simulink model "ODE_neurospora_model_leloup"  (R2015a)
settings: Solver=ode4  StartTime=0.0  StopTime=72  FixedStep=0.01  RelTol=1e-3
values from neighbouring files (symbols this model uses):
  daynight_on = 0    [ALL_neurospora_init.m]    (also in ALL_neurospora_sim_run.m; FUZZY_deg_neurospora_init.m; FUZZY_deg_neurospora_sim_run.m; FUZZY_tsc_neurospora_init.m)
  k_1 = 0.5    [ALL_neurospora_init.m]    (also in FUZZY_deg_neurospora_init.m; FUZZY_tsc_neurospora_init.m; FUZZY_tsc_tsl_neurospora_init.m; FUZZY_tsl_neurospora_init.m)
  k_2 = 0.6    [ALL_neurospora_init.m]    (also in FUZZY_deg_neurospora_init.m; FUZZY_tsc_neurospora_init.m; FUZZY_tsc_tsl_neurospora_init.m; FUZZY_tsl_neurospora_init.m)
  K_d = 0.13    [ALL_neurospora_init.m]    (also in FUZZY_deg_neurospora_init.m; FUZZY_tsc_neurospora_init.m; FUZZY_tsc_tsl_neurospora_init.m; FUZZY_tsl_neurospora_init.m)
  K_I = 1    [ALL_neurospora_init.m]    (also in FUZZY_deg_neurospora_init.m; FUZZY_tsc_neurospora_init.m; FUZZY_tsc_tsl_neurospora_init.m; FUZZY_tsl_neurospora_init.m)
  K_m = 0.5    [ALL_neurospora_init.m]    (also in FUZZY_deg_neurospora_init.m; FUZZY_tsc_neurospora_init.m; FUZZY_tsc_tsl_neurospora_init.m; FUZZY_tsl_neurospora_init.m)
  k_s = 0.5    [ALL_neurospora_init.m]    (also in FUZZY_deg_neurospora_init.m; FUZZY_tsc_neurospora_init.m; FUZZY_tsc_tsl_neurospora_init.m; FUZZY_tsl_neurospora_init.m)
  n = 4    [ALL_neurospora_init.m]    (also in FUZZY_deg_neurospora_init.m; FUZZY_tsc_neurospora_init.m; FUZZY_tsc_tsl_neurospora_init.m; FUZZY_tsl_neurospora_init.m)
  v_d = 1.4    [ALL_neurospora_init.m]    (also in FUZZY_deg_neurospora_init.m; FUZZY_tsc_neurospora_init.m; FUZZY_tsc_tsl_neurospora_init.m; FUZZY_tsl_neurospora_init.m)
  v_m = 0.505    [ALL_neurospora_init.m]    (also in FUZZY_deg_neurospora_init.m; FUZZY_tsc_neurospora_init.m; FUZZY_tsc_tsl_neurospora_init.m; FUZZY_tsl_neurospora_init.m)
settings Model: Creator=jureb  LastModifiedBy=jureb

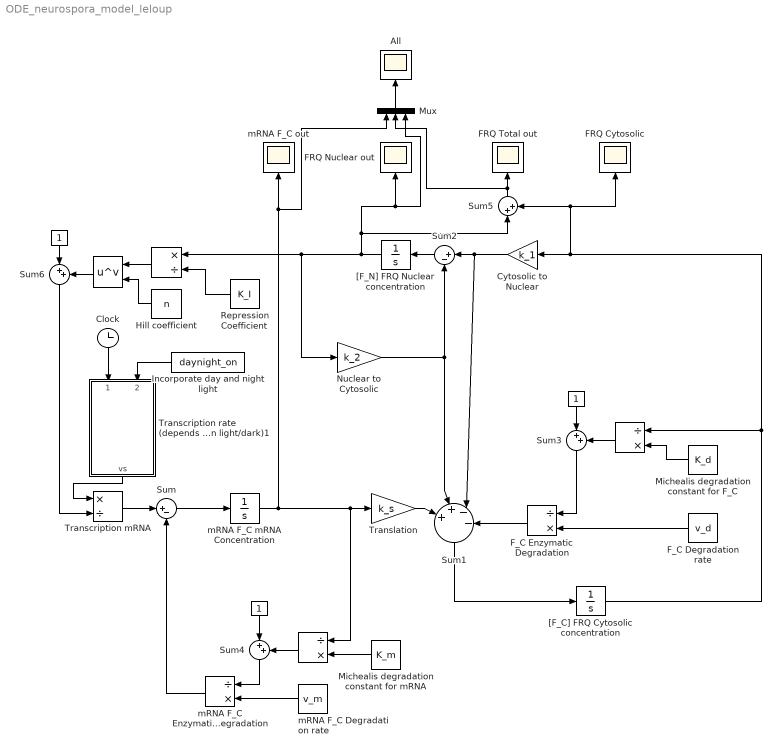
== system ODE_neurospora_model_leloup ==
  " " : Math  Operator=pow  SaturateOnIntegerOverflow=on
  " " : Product  Inputs=/*
  " " : Product  Inputs=*/
  "          " : Constant
  " " : Constant
  " " : Constant
  " " : Product  Inputs=/*
  All : Scope
      settings: TimeRange=71.999776  YMin=0  YMax=9  SaveName=All
  Clock : Clock
  Cytosolic to Nuclear : Gain  Gain=k_1
  FRQ Cytosolic : Scope
      settings: TimeRange=71.999776  YMin=0.5  YMax=10  SaveName=FC_ODE
  FRQ Nuclear out : Scope
      settings: TimeRange=71.999776  YMin=0  YMax=4.5  SaveName=F_N
  FRQ Total out : Scope
      settings: TimeRange=71.999776  YMin=0.5  YMax=10  SaveName=F_ODE
  F_C Degradation rate : Constant  Value=v_d
  F_C Enzymatic Degradation : Product  Inputs=/*
  Hill coefficient : Constant  Value=n
  Incorporate day and night light : Constant  Value=daynight_on
  Michealis degradation constant for F_C : Constant  Value=K_d
  Michealis degradation constant for mRNA : Constant  Value=K_m
  Mux : Mux  Inputs=3
  Nuclear to Cytosolic : Gain  Gain=k_2
  Repression Coefficient : Constant  Value=K_I
  Sum : Sum  Inputs=|+-
  Sum1 : Sum  Inputs=|+|+|-|-
  Sum2 : Sum  Inputs=|+-
  Sum{3..6} (4 alike) : Sum  Inputs=|++
  Transcription mRNA : Product  Inputs=*/
  Transcription rate (depends on light/dark)1 : MATLAB Function  TreatAsAtomicUnit=on
  Translation : Gain  Gain=k_s
  "[F_C] FRQ Cytosolic concentration " : Integrator  InitialCondition=1
  "[F_N] FRQ Nuclear concentration" : Integrator  InitialCondition=1
  mRNA F_C Degradation rate : Constant  Value=v_m
  mRNA F_C Enzymatic Degradation : Product  Inputs=/*
  mRNA F_C mRNA Concentration : Integrator  InitialCondition=1
  mRNA F_C out : Scope
      settings: TimeRange=71.999776  YMin=0  YMax=6  SaveName=mRNA
  wires:
  Sum6/1 -> Transcription mRNA/2
  "          "/1 -> Sum6/1
  " "/1 -> Sum6/2
  Hill coefficient/1 -> " "/2
  Sum/1 -> mRNA F_C mRNA Concentration/1
  " "/1 -> " "/1
  mRNA F_C mRNA Concentration/1 -> Mux/1, mRNA F_C out/1, " "/1, Translation/1
  mRNA F_C Enzymatic Degradation/1 -> Sum/2
  "[F_N] FRQ Nuclear concentration"/1 -> " "/1, Nuclear to Cytosolic/1, Mux/3, FRQ Nuclear out/1, Sum5/1
  Repression Coefficient/1 -> " "/2
  Sum1/1 -> "[F_C] FRQ Cytosolic concentration "/1
  Cytosolic to Nuclear/1 -> Sum1/3, Sum2/1
  Sum2/1 -> "[F_N] FRQ Nuclear concentration"/1
  Nuclear to Cytosolic/1 -> Sum1/2, Sum2/2
  mRNA F_C Degradation rate/1 -> mRNA F_C Enzymatic Degradation/2
  " "/1 -> Sum4/1
  " "/1 -> Sum4/2
  Michealis degradation constant for mRNA/1 -> " "/2
  Sum4/1 -> mRNA F_C Enzymatic Degradation/1
  "[F_C] FRQ Cytosolic concentration "/1 -> FRQ Cytosolic/1, Sum5/2, Cytosolic to Nuclear/1, " "/1
  F_C Enzymatic Degradation/1 -> Sum1/4
  F_C Degradation rate/1 -> F_C Enzymatic Degradation/2
  " "/1 -> Sum3/1
  " "/1 -> Sum3/2
  Michealis degradation constant for F_C/1 -> " "/2
  Sum3/1 -> F_C Enzymatic Degradation/1
  Translation/1 -> Sum1/1
  Mux/1 -> All/1
  Clock/1 -> Transcription rate (depends on light/dark)1/1(sim_time)
  Transcription rate (depends on light/dark)1/1(vs) -> Transcription mRNA/1
  Incorporate day and night light/1 -> Transcription rate (depends on light/dark)1/2(daynight_on)
  Sum5/1 -> Mux/2, FRQ Total out/1
  Transcription mRNA/1 -> Sum/1

== matlab function ODE_neurospora_model_leloup/Transcription rate (depends on light//dark)1 ==
  data: sim_time input; vs output; daynight_on input
function vs = day_night(sim_time,daynight_on)

vs_day = 2;
vs_night = 1.6;

if daynight_on == 1
    if ((sim_time > 0 && sim_time < 12) || (sim_time > 24 && sim_time < 36) || (sim_time > 48 && sim_time < 60)) % DAY
        vs = vs_day;
    else % NIGHT
        vs = vs_night;
    end
else % NO DIFFERENTIATION BETWEEN NIGHT AND DAY
    vs = vs_night;
end
